simulink model "bosy_subsystem"  (R2017b)
settings: Solver=VariableStepAuto  StartTime=0.0  StopTime=10.0  RelTol=1e-3
undefined symbols (not defined in the file): g, m1
settings Model: Creator=jc2182  LastModifiedBy=jc2182

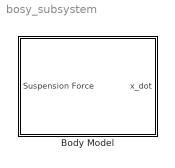
== system bosy_subsystem ==
  Body Model : Subsystem

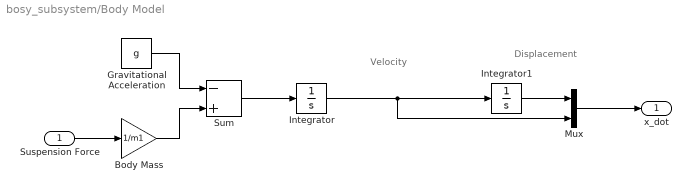
== system bosy_subsystem/Body Model ==
  note: Displacement
  note: Velocity
  Suspension Force : Inport
  Body Mass : Gain  Gain=1/m1
  Gravitational Acceleration : Constant  Value=g
  Integrator : Integrator
  Integrator1 : Integrator
  Mux : Mux  Inputs=2
  Sum : Sum  Inputs=-+
  x_dot : Outport
  wires:
  Integrator/1 -> Mux/2, Integrator1/1
  Sum/1 -> Integrator/1
  Gravitational Acceleration/1 -> Sum/1
  Mux/1 -> x_dot/1
  Suspension Force/1 -> Body Mass/1
  Body Mass/1 -> Sum/2
  Integrator1/1 -> Mux/1
